simulink model "regcontrol_model_3ph"  (R2018b)
settings: Solver=VariableStepAuto  StartTime=0.0  StopTime=10.0  RelTol=1e-3
values from neighbouring files (symbols this model uses):
  BandWidth = Simulink.Parameter    [start.m]
  BaseVoltage = Simulink.Parameter    [start.m]
  CogenEnabled = false    [regcontrol_emulator.m]    (also in start.m = Simulink.Parameter)
  ElementTerminal = 0    [start.m]
  FPTphase = Simulink.Parameter(FPTphases.DEFAULT)    [regcontrol_emulator.m]    (also in start.m = 1)
  InCogenMode = false    [regcontrol_emulator.m]
  InReverseMode = false    [regcontrol_emulator.m]
  IsReversible = Simulink.Parameter    [start.m]
  LastHandle = RecentExecuted(1,NewCtrlQueueFields.Handle, end)    [LogEvent_1ph.m]    (also in LogEvent_1ph_old.m)
  LDC_Z = Simulink.Parameter    [start.m]
  MaxTap = 1.10    (= 1.1)    [Transformer.m]
  MinTap = 0.90    (= 0.9)    [Transformer.m]
  PTratio = Simulink.Parameter    [start.m]
  R = 0    [start.m]
  RevBand = Simulink.Parameter    [start.m]
  RevVreg = Simulink.Parameter    [start.m]
  TapLimitPerChange = Simulink.Parameter    [start.m]
  UsingRegulatedBus = Simulink.Parameter    [start.m]
  Vlimit = Simulink.Parameter    [start.m]
  Vreg = Simulink.Parameter    [start.m]
  X = 0    [start.m]
undefined symbols (not defined in the file or in its folder): Armed, ControlledTransformerConnection, ControlledTransformerCurrents, ControlledTransformerPowers, ControlledTransformerVoltages, CTRating, DeltaDirection, IsInverseTime, LastQueue, LookingForward, m, n, NumConductors, NumPhases, PresentTap, RevBackHandle, RevDelay, ReversePending, RevHandle, revLDC_Z, RevPowerThreshold, revR, revX, TapDelay, TapIncrement, TapWinding, TimeDelay, TimeInSec, VTerminal
(part 1 of 4)
settings Model: Creator=Michael Girbino  LastModifiedBy=Michael Girbino
settings DebuggingCC: LibraryContextMissingDiagnostic=none
settings SFSimCC: SimUseLocalCustomCode=off
settings RTWCC: RTWUseLocalCustomCode=off
settings CodeAppCC: StateflowObjectComments=on

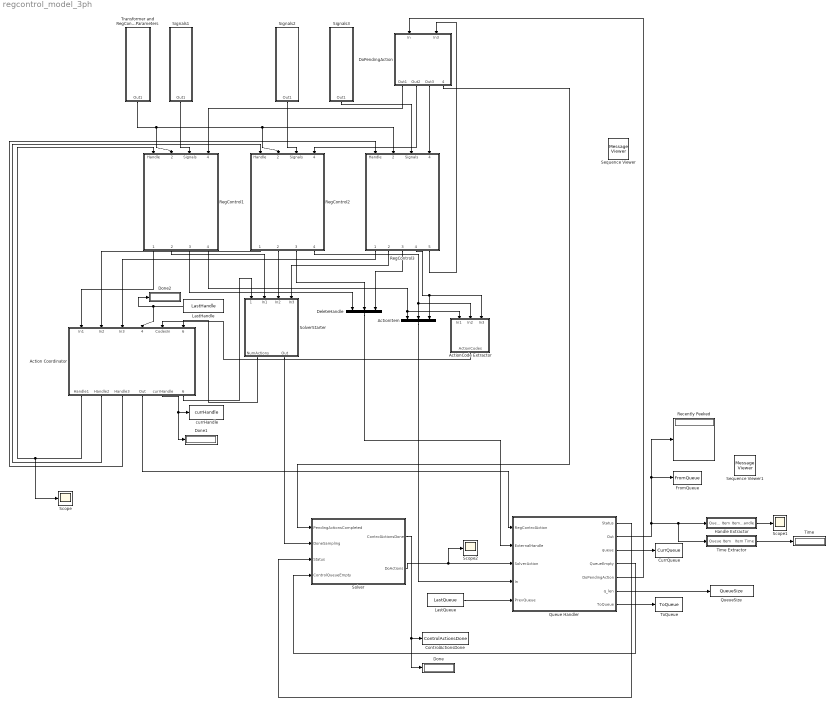
== system regcontrol_model_3ph ==
  Action Coordinator : Stateflow chart  TreatAsAtomicUnit=on
  "ActionCode Extractor " : Subsystem
  ActionItem : Concatenate  NumInputs=3  Mode=Multidimensional array  ConcatenateDimension=2
  ControlActionsDone : ToWorkspace  VariableName=ControlActionsDone  SaveFormat=Timeseries  SampleTime=-1
      settings: MaxDataPoints=1
  CurrQueue : ToWorkspace  VariableName=CurrQueue  SaveFormat=Structure With Time  SampleTime=1
  DeleteHandle : Mux  Inputs=3
  DoPendingAction : Stateflow chart  TreatAsAtomicUnit=on
  Done : Display
  Done1 : Display
  Done2 : Display
  FromQueue : ToWorkspace  VariableName=FromQueue  SaveFormat=Structure With Time  SampleTime=1
  Handle Extractor : Subsystem
  LastHandle : Constant  Value=LastHandle
  LastQueue : Constant  Value=LastQueue  VectorParams1D=off  OutDataTypeStr=double
  Queue Handler : Stateflow chart  TreatAsAtomicUnit=on
  QueueSize : ToWorkspace  VariableName=QueueSize  SaveFormat=Timeseries  SampleTime=-1
      settings: MaxDataPoints=1
  Recently Peeked : Display
  RegControl1 : Subsystem
  RegControl2 : Subsystem
  RegControl3 : Subsystem
  Scope : Scope
  Scope1 : Scope
  Scope2 : Scope
  Sequence Viewer : MessageViewer
  Sequence Viewer1 : MessageViewer
  Signals1 : Subsystem
  Signals2 : Subsystem
  Signals3 : Subsystem
  Solver : Stateflow chart  TreatAsAtomicUnit=on
  SolverStarter : Stateflow chart  TreatAsAtomicUnit=on
  Time : Display
  Time Extractor : Subsystem
  ToQueue : ToWorkspace  VariableName=ToQueue  SaveFormat=Structure With Time  SampleTime=-1
      settings: MaxDataPoints=1
  Transformer and RegControl Parameters : Subsystem
  currHandle : ToWorkspace  VariableName=currHandle  SaveFormat=Timeseries  SampleTime=-1
      settings: MaxDataPoints=1
  wires:
  Signals1/1(Out1) -> RegControl1/3(Signals)
  Transformer and RegControl Parameters/1(Out1) -> RegControl3/2(Equipment), RegControl2/2(Equipment), RegControl1/2(Equipment)
  DoPendingAction/1(Out1) -> RegControl1/4(DoPendingAction)
  DoPendingAction/2(Out2) -> RegControl2/4(DoPendingAction)
  DoPendingAction/3(Out3) -> RegControl3/4(DoPendingAction)
  RegControl1/1(DoActions) -> Action Coordinator/1(In1)
  RegControl2/1(DoActions) -> Action Coordinator/2(In2)
  RegControl3/1(DoActions) -> Action Coordinator/3(In3)
  RegControl1/2(DoneSampling) -> SolverStarter/2(In1)
  RegControl2/2(DoneSampling) -> SolverStarter/3(In2)
  RegControl3/2(DoneSampling) -> SolverStarter/4(In3)
  RegControl1/3(DeleteHandle) -> DeleteHandle/1
  RegControl2/3(DeleteHandle) -> DeleteHandle/2
  RegControl3/3(DeleteHandle) -> DeleteHandle/3
  RegControl2/4(ActionItem) -> "ActionCode Extractor "/2(In2), ActionItem/2
  RegControl3/4(ActionItem) -> "ActionCode Extractor "/3(In3), ActionItem/3
  DeleteHandle/1 -> Queue Handler/2(ExternalHandle)
  Queue Handler/6(q_len) -> QueueSize/1
  Solver/2(DoActions) -> Scope2/1, Queue Handler/3(SolverAction)
  Handle Extractor/1(Item Handle) -> Scope1/1
  Action Coordinator/4(Out) -> Queue Handler/1(RegControlAction)
  SolverStarter/2(Out) -> Solver/2(DoneSampling)
  Queue Handler/2(Out) -> Time Extractor/1(Queue Item), Handle Extractor/1(Queue Item), FromQueue/1, Recently Peeked/1
  Queue Handler/5(DoPendingAction) -> DoPendingAction/1(In)
  Queue Handler/4(QueueEmpty) -> Solver/4(ControlQueueEmpty)
  Time Extractor/1(Item Time) -> Time/1
  Queue Handler/3(queue) -> CurrQueue/1
  LastQueue/1 -> Queue Handler/5(PrevQueue)
  Solver/1(ControlActionsDone) -> Done/1, ControlActionsDone/1
  ActionItem/1 -> Queue Handler/4(In)
  Queue Handler/1(Status) -> Solver/3(Status)
  Signals2/1(Out1) -> RegControl2/3(Signals)
  Signals3/1(Out1) -> RegControl3/3(Signals)
  Action Coordinator/5(currHandle) -> Done1/1, currHandle/1
  LastHandle/1 -> Done2/1, Action Coordinator/4(LastHandle)
  Action Coordinator/1(Handle1) -> Scope/1, RegControl1/1(Handle)
  Action Coordinator/2(Handle2) -> RegControl2/1(Handle)
  Action Coordinator/3(Handle3) -> RegControl3/1(Handle)
  Queue Handler/7(ToQueue) -> ToQueue/1
  "ActionCode Extractor "/1(ActionCodes) -> Action Coordinator/5(CodesIn)
  RegControl1/4(ActionItem) -> "ActionCode Extractor "/1(In1), ActionItem/1
  Action Coordinator/6(ActionsDone) -> SolverStarter/1(ActionsDone)
  SolverStarter/1(NumActions) -> Action Coordinator/6(NumActions)
  DoPendingAction/4(PendingActionsCompleted) -> Solver/1(PendingActionsCompleted)
  RegControl3/5(PendingActionCompleted) -> DoPendingAction/2(In3)

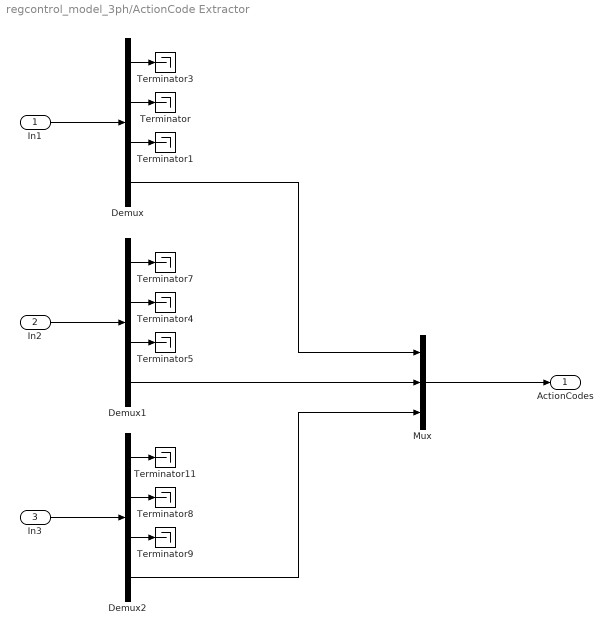
== system regcontrol_model_3ph/ActionCode Extractor  ==
  In1 : Inport
  In2 : Inport  Port=2
  In3 : Inport  Port=3
  Demux : Demux
  Demux1 : Demux
  Demux2 : Demux
  Mux : Mux  Inputs=3
  Terminator{,1,3..5,7..9,11} (9 alike) : Terminator
  ActionCodes : Outport
  wires:
  In1/1 -> Demux/1
  Demux/3 -> Terminator1/1
  Demux/4 -> Mux/1
  Demux/1 -> Terminator3/1
  Demux/2 -> Terminator/1
  Demux1/2 -> Terminator4/1
  Demux1/1 -> Terminator7/1
  Demux1/4 -> Mux/2
  Demux1/3 -> Terminator5/1
  In2/1 -> Demux1/1
  In3/1 -> Demux2/1
  Demux2/3 -> Terminator9/1
  Demux2/4 -> Mux/3
  Demux2/1 -> Terminator11/1
  Demux2/2 -> Terminator8/1
  Mux/1 -> ActionCodes/1

== system regcontrol_model_3ph/Handle Extractor ==
  Queue Item : Inport
  Demux : Demux  Outputs=6
  Terminator{,1..4} (5 alike) : Terminator
  Item Handle : Outport
  wires:
  Queue Item/1 -> Demux/1
  Demux/4 -> Terminator2/1
  Demux/3 -> Terminator1/1
  Demux/5 -> Terminator3/1
  Demux/1 -> Item Handle/1
  Demux/2 -> Terminator/1
  Demux/6 -> Terminator4/1

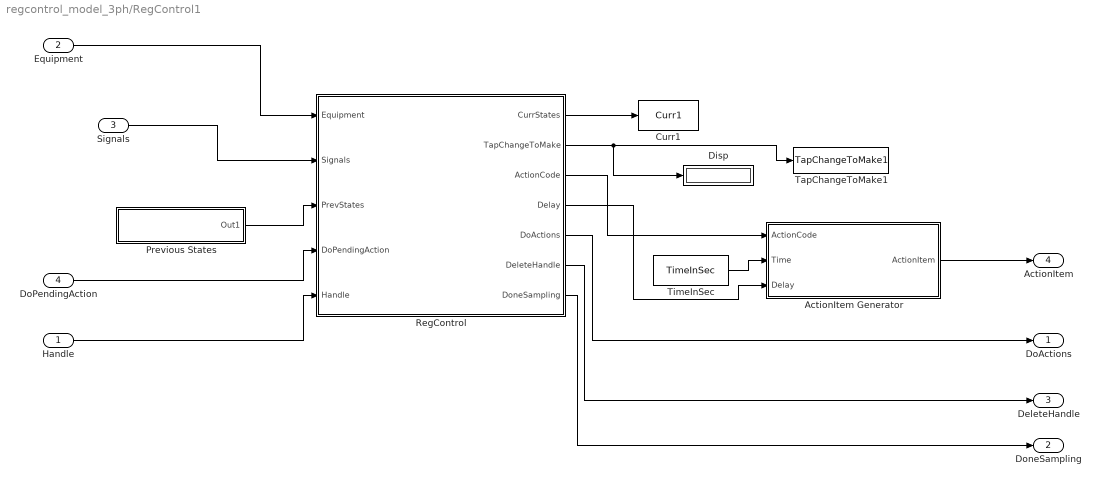
== system regcontrol_model_3ph/RegControl1 ==
  Handle : Inport
  Equipment : Inport  Port=2
  Signals : Inport  Port=3
  DoPendingAction : Inport  Port=4
  ActionItem Generator : Subsystem
  Curr1 : ToWorkspace  VariableName=Curr1  SaveFormat=Timeseries  SampleTime=-1
      settings: MaxDataPoints=1
  Disp : Display
  Previous States : Subsystem
  RegControl : Stateflow chart  TreatAsAtomicUnit=on
  TapChangeToMake1 : ToWorkspace  VariableName=TapChangeToMake1  SaveFormat=Timeseries  SampleTime=-1
      settings: MaxDataPoints=1
  TimeInSec : Constant  Value=TimeInSec  OutDataTypeStr=double
  DoActions : Outport
  DoneSampling : Outport  Port=2
  DeleteHandle : Outport  Port=3
  ActionItem : Outport  Port=4
  wires:
  RegControl/5(DoActions) -> DoActions/1
  RegControl/2(TapChangeToMake) -> Disp/1, TapChangeToMake1/1
  RegControl/4(Delay) -> ActionItem Generator/3(Delay)
  RegControl/3(ActionCode) -> ActionItem Generator/1(ActionCode)
  TimeInSec/1 -> ActionItem Generator/2(Time)
  ActionItem Generator/1(ActionItem) -> ActionItem/1
  RegControl/1(CurrStates) -> Curr1/1
  DoPendingAction/1 -> RegControl/4(DoPendingAction)
  Equipment/1 -> RegControl/1(Equipment)
  Signals/1 -> RegControl/2(Signals)
  RegControl/7(DoneSampling) -> DoneSampling/1
  Previous States/1(Out1) -> RegControl/3(PrevStates)
  RegControl/6(DeleteHandle) -> DeleteHandle/1
  Handle/1 -> RegControl/5(Handle)

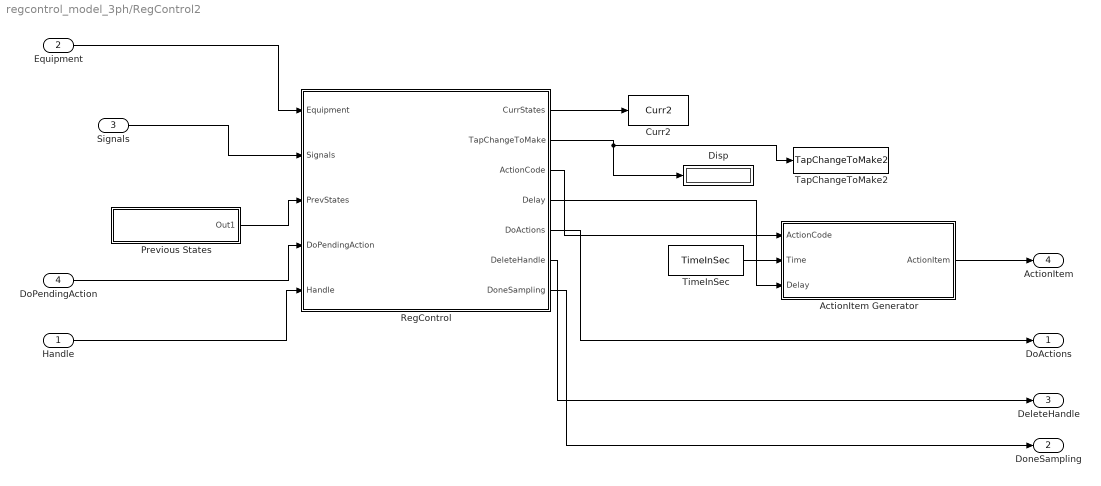
== system regcontrol_model_3ph/RegControl2 ==
  Handle : Inport
  Equipment : Inport  Port=2
  Signals : Inport  Port=3
  DoPendingAction : Inport  Port=4
  ActionItem Generator : Subsystem
  Curr2 : ToWorkspace  VariableName=Curr2  SaveFormat=Timeseries  SampleTime=-1
      settings: MaxDataPoints=1
  Disp : Display
  Previous States : Subsystem
  RegControl : Stateflow chart  TreatAsAtomicUnit=on
  TapChangeToMake2 : ToWorkspace  VariableName=TapChangeToMake2  SaveFormat=Timeseries  SampleTime=-1
      settings: MaxDataPoints=1
  TimeInSec : Constant  Value=TimeInSec  OutDataTypeStr=double
  DoActions : Outport
  DoneSampling : Outport  Port=2
  DeleteHandle : Outport  Port=3
  ActionItem : Outport  Port=4
  wires:
  RegControl/6(DeleteHandle) -> DeleteHandle/1
  Previous States/1(Out1) -> RegControl/3(PrevStates)
  RegControl/7(DoneSampling) -> DoneSampling/1
  Signals/1 -> RegControl/2(Signals)
  Equipment/1 -> RegControl/1(Equipment)
  DoPendingAction/1 -> RegControl/4(DoPendingAction)
  RegControl/1(CurrStates) -> Curr2/1
  ActionItem Generator/1(ActionItem) -> ActionItem/1
  TimeInSec/1 -> ActionItem Generator/2(Time)
  RegControl/3(ActionCode) -> ActionItem Generator/1(ActionCode)
  RegControl/4(Delay) -> ActionItem Generator/3(Delay)
  RegControl/2(TapChangeToMake) -> TapChangeToMake2/1, Disp/1
  RegControl/5(DoActions) -> DoActions/1
  Handle/1 -> RegControl/5(Handle)

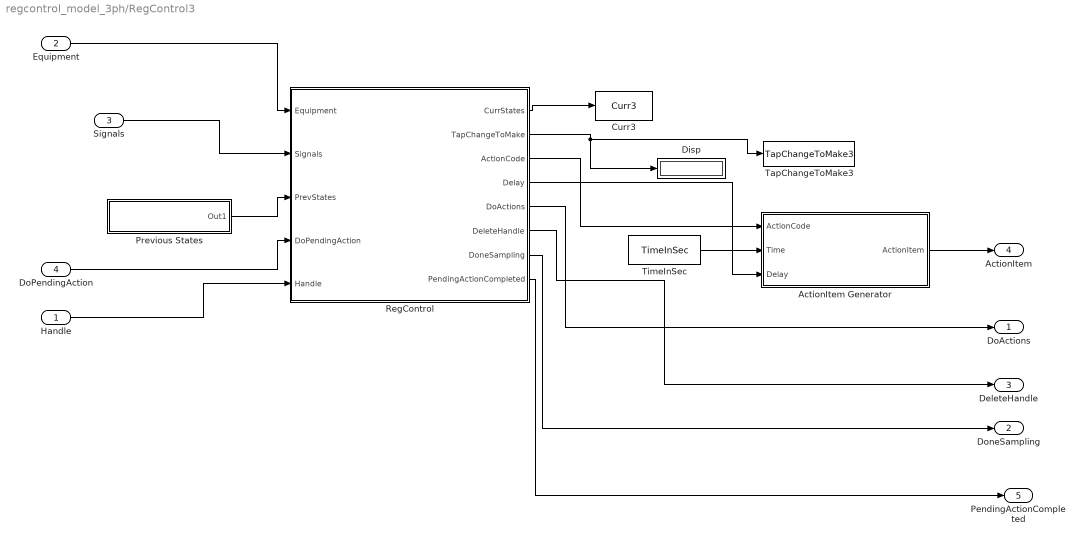
== system regcontrol_model_3ph/RegControl3 ==
  Handle : Inport
  Equipment : Inport  Port=2
  Signals : Inport  Port=3
  DoPendingAction : Inport  Port=4
  ActionItem Generator : Subsystem
  Curr3 : ToWorkspace  VariableName=Curr3  SaveFormat=Timeseries  SampleTime=-1
      settings: MaxDataPoints=1
  Disp : Display
  Previous States : Subsystem
  RegControl : Stateflow chart  TreatAsAtomicUnit=on
  TapChangeToMake3 : ToWorkspace  VariableName=TapChangeToMake3  SaveFormat=Timeseries  SampleTime=-1
      settings: MaxDataPoints=1
  TimeInSec : Constant  Value=TimeInSec  OutDataTypeStr=double
  DoActions : Outport
  DoneSampling : Outport  Port=2
  DeleteHandle : Outport  Port=3
  ActionItem : Outport  Port=4
  PendingActionCompleted : Outport  Port=5
  wires:
  RegControl/5(DoActions) -> DoActions/1
  RegControl/2(TapChangeToMake) -> Disp/1, TapChangeToMake3/1
  RegControl/4(Delay) -> ActionItem Generator/3(Delay)
  RegControl/3(ActionCode) -> ActionItem Generator/1(ActionCode)
  TimeInSec/1 -> ActionItem Generator/2(Time)
  ActionItem Generator/1(ActionItem) -> ActionItem/1
  RegControl/1(CurrStates) -> Curr3/1
  DoPendingAction/1 -> RegControl/4(DoPendingAction)
  Equipment/1 -> RegControl/1(Equipment)
  Signals/1 -> RegControl/2(Signals)
  RegControl/7(DoneSampling) -> DoneSampling/1
  Previous States/1(Out1) -> RegControl/3(PrevStates)
  RegControl/6(DeleteHandle) -> DeleteHandle/1
  Handle/1 -> RegControl/5(Handle)
  RegControl/8(PendingActionCompleted) -> PendingActionCompleted/1

== system regcontrol_model_3ph/Signals1 ==
  Bus Creator1 : BusCreator  Inputs=4  OutDataTypeStr=Bus: SignalBus
      settings: InheritFromInputs=off
  ControlledTransformerCurrents : Constant  Value=ControlledTransformerCurrents(:,1)
  ControlledTransformerPowers : Constant  Value=ControlledTransformerPowers(:,1)
  ControlledTransformerVoltages : Constant  Value=ControlledTransformerVoltages(:,1)
  VTerminal : Constant  Value=VTerminal(:,1)
  Out1 : Outport
  wires:
  Bus Creator1/1 -> Out1/1
  ControlledTransformerPowers/1 -> Bus Creator1/3
  ControlledTransformerVoltages/1 -> Bus Creator1/1
  ControlledTransformerCurrents/1 -> Bus Creator1/2
  VTerminal/1 -> Bus Creator1/4

== system regcontrol_model_3ph/Signals2 ==
  Bus Creator1 : BusCreator  Inputs=4  OutDataTypeStr=Bus: SignalBus
      settings: InheritFromInputs=off
  ControlledTransformerCurrents : Constant  Value=ControlledTransformerCurrents(:,2)
  ControlledTransformerPowers : Constant  Value=ControlledTransformerPowers(:,2)
  ControlledTransformerVoltages : Constant  Value=ControlledTransformerVoltages(:,2)
  VTerminal : Constant  Value=VTerminal(:,2)
  Out1 : Outport
  wires:
  ControlledTransformerCurrents/1 -> Bus Creator1/2
  ControlledTransformerPowers/1 -> Bus Creator1/3
  VTerminal/1 -> Bus Creator1/4
  ControlledTransformerVoltages/1 -> Bus Creator1/1
  Bus Creator1/1 -> Out1/1

== system regcontrol_model_3ph/Signals3 ==
  Bus Creator1 : BusCreator  Inputs=4  OutDataTypeStr=Bus: SignalBus
      settings: InheritFromInputs=off
  ControlledTransformerCurrents : Constant  Value=ControlledTransformerCurrents(:,3)
  ControlledTransformerPowers : Constant  Value=ControlledTransformerPowers(:,3)
  ControlledTransformerVoltages : Constant  Value=ControlledTransformerVoltages(:,3)
  VTerminal : Constant  Value=VTerminal(:,3)
  Out1 : Outport
  wires:
  ControlledTransformerCurrents/1 -> Bus Creator1/2
  ControlledTransformerPowers/1 -> Bus Creator1/3
  VTerminal/1 -> Bus Creator1/4
  ControlledTransformerVoltages/1 -> Bus Creator1/1
  Bus Creator1/1 -> Out1/1

== system regcontrol_model_3ph/Time Extractor ==
  Queue Item : Inport
  Demux : Demux  Outputs=6
  Terminator{,1..4} (5 alike) : Terminator
  Item Time : Outport
  wires:
  Demux/5 -> Terminator3/1
  Demux/3 -> Terminator1/1
  Demux/4 -> Terminator2/1
  Demux/1 -> Terminator/1
  Demux/2 -> Item Time/1
  Queue Item/1 -> Demux/1
  Demux/6 -> Terminator4/1

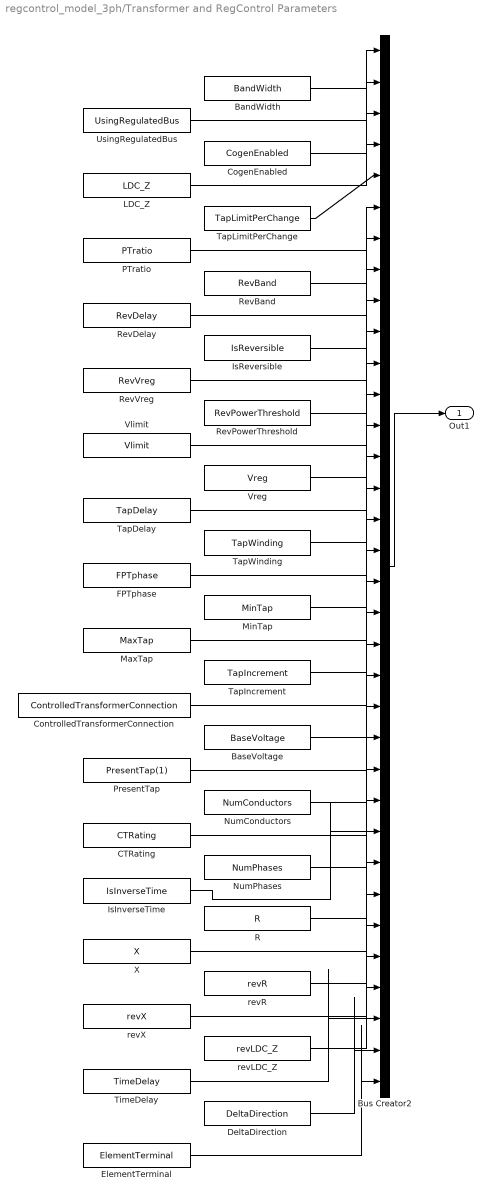
== system regcontrol_model_3ph/Transformer and RegControl Parameters ==
  BandWidth : Constant  Value=BandWidth
  BaseVoltage : Constant  Value=BaseVoltage
  Bus Creator2 : BusCreator  Inputs=34  OutDataTypeStr=Bus: EquipmentBus
      settings: InheritFromInputs=off
  CTRating : Constant  Value=CTRating
  CogenEnabled : Constant  Value=CogenEnabled
  ControlledTransformerConnection : Constant  Value=ControlledTransformerConnection
  DeltaDirection : Constant  Value=DeltaDirection
  ElementTerminal : Constant  Value=ElementTerminal
  FPTphase : Constant  Value=FPTphase
  IsInverseTime : Constant  Value=IsInverseTime
  IsReversible : Constant  Value=IsReversible
  LDC_Z : Constant  Value=LDC_Z
  MaxTap : Constant  Value=MaxTap
  MinTap : Constant  Value=MinTap
  NumConductors : Constant  Value=NumConductors
  NumPhases : Constant  Value=NumPhases
  PTratio : Constant  Value=PTratio
  PresentTap : Constant  Value=PresentTap(1)
  R : Constant  Value=R
  RevBand : Constant  Value=RevBand
  RevDelay : Constant  Value=RevDelay
  RevPowerThreshold : Constant  Value=RevPowerThreshold
  RevVreg : Constant  Value=RevVreg
  TapDelay : Constant  Value=TapDelay
  TapIncrement : Constant  Value=TapIncrement
  TapLimitPerChange : Constant  Value=TapLimitPerChange
  TapWinding : Constant  Value=TapWinding
  TimeDelay : Constant  Value=TimeDelay
  UsingRegulatedBus : Constant  Value=UsingRegulatedBus
  Vlimit : Constant  Value=Vlimit
  Vreg : Constant  Value=Vreg
  X : Constant  Value=X
  revLDC_Z : Constant  Value=revLDC_Z
  revR : Constant  Value=revR
  revX : Constant  Value=revX
  Out1 : Outport
  wires:
  UsingRegulatedBus/1 -> Bus Creator2/2
  BandWidth/1 -> Bus Creator2/1
  TapWinding/1 -> Bus Creator2/15
  TapDelay/1 -> Bus Creator2/14
  Vreg/1 -> Bus Creator2/13
  Vlimit/1 -> Bus Creator2/12
  RevPowerThreshold/1 -> Bus Creator2/11
  RevVreg/1 -> Bus Creator2/10
  IsReversible/1 -> Bus Creator2/9
  RevDelay/1 -> Bus Creator2/8
  RevBand/1 -> Bus Creator2/7
  PTratio/1 -> Bus Creator2/6
  TapLimitPerChange/1 -> Bus Creator2/5
  LDC_Z/1 -> Bus Creator2/4
  CogenEnabled/1 -> Bus Creator2/3
  Bus Creator2/1 -> Out1/1
  FPTphase/1 -> Bus Creator2/16
  MinTap/1 -> Bus Creator2/17
  MaxTap/1 -> Bus Creator2/18
  TapIncrement/1 -> Bus Creator2/19
  ControlledTransformerConnection/1 -> Bus Creator2/20
  BaseVoltage/1 -> Bus Creator2/21
  PresentTap/1 -> Bus Creator2/22
  NumConductors/1 -> Bus Creator2/23
  CTRating/1 -> Bus Creator2/24
  NumPhases/1 -> Bus Creator2/25
  revLDC_Z/1 -> Bus Creator2/31
  revX/1 -> Bus Creator2/30
  revR/1 -> Bus Creator2/29
  X/1 -> Bus Creator2/28
  R/1 -> Bus Creator2/27
  IsInverseTime/1 -> Bus Creator2/26
  TimeDelay/1 -> Bus Creator2/32
  DeltaDirection/1 -> Bus Creator2/33
  ElementTerminal/1 -> Bus Creator2/34

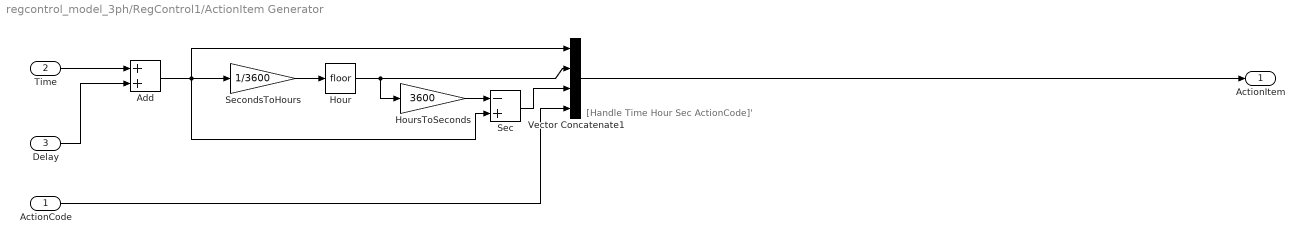
== system regcontrol_model_3ph/RegControl1/ActionItem Generator ==
  note: [Handle Time Hour Sec ActionCode]'
  ActionCode : Inport
  Time : Inport  Port=2
  Delay : Inport  Port=3
  Add : Sum
  Hour : Rounding
  HoursToSeconds : Gain  Gain=3600
  Sec : Sum  Inputs=-+
  SecondsToHours : Gain  Gain=1/3600
  Vector Concatenate1 : Concatenate  NumInputs=4
  ActionItem : Outport
  wires:
  Time/1 -> Add/1
  Hour/1 -> Vector Concatenate1/2, HoursToSeconds/1
  SecondsToHours/1 -> Hour/1
  Vector Concatenate1/1 -> ActionItem/1
  HoursToSeconds/1 -> Sec/1
  Sec/1 -> Vector Concatenate1/3
  ActionCode/1 -> Vector Concatenate1/4
  Delay/1 -> Add/2
  Add/1 -> Vector Concatenate1/1, Sec/2, SecondsToHours/1

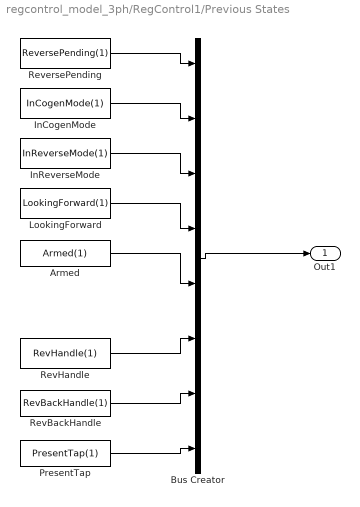
== system regcontrol_model_3ph/RegControl1/Previous States ==
  Armed : Constant  Value=Armed(1)
  Bus Creator : BusCreator  Inputs=8  OutDataTypeStr=Bus: StatesBus
      settings: InheritFromInputs=off
  InCogenMode : Constant  Value=InCogenMode(1)
  InReverseMode : Constant  Value=InReverseMode(1)
  LookingForward : Constant  Value=LookingForward(1)
  PresentTap : Constant  Value=PresentTap(1)
  RevBackHandle : Constant  Value=RevBackHandle(1)
  RevHandle : Constant  Value=RevHandle(1)
  ReversePending : Constant  Value=ReversePending(1)
  Out1 : Outport
  wires:
  Bus Creator/1 -> Out1/1
  ReversePending/1 -> Bus Creator/1
  InCogenMode/1 -> Bus Creator/2
  InReverseMode/1 -> Bus Creator/3
  LookingForward/1 -> Bus Creator/4
  Armed/1 -> Bus Creator/5
  RevHandle/1 -> Bus Creator/6
  RevBackHandle/1 -> Bus Creator/7
  PresentTap/1 -> Bus Creator/8

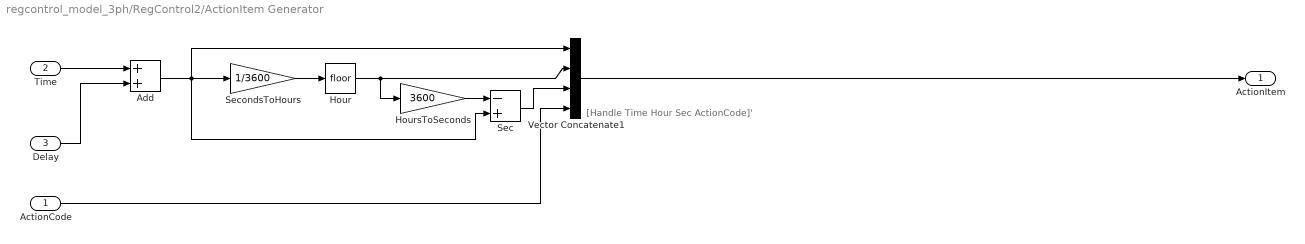
== system regcontrol_model_3ph/RegControl2/ActionItem Generator ==
  note: [Handle Time Hour Sec ActionCode]'
  ActionCode : Inport
  Time : Inport  Port=2
  Delay : Inport  Port=3
  Add : Sum
  Hour : Rounding
  HoursToSeconds : Gain  Gain=3600
  Sec : Sum  Inputs=-+
  SecondsToHours : Gain  Gain=1/3600
  Vector Concatenate1 : Concatenate  NumInputs=4
  ActionItem : Outport
  wires:
  Delay/1 -> Add/2
  Add/1 -> Vector Concatenate1/1, Sec/2, SecondsToHours/1
  HoursToSeconds/1 -> Sec/1
  SecondsToHours/1 -> Hour/1
  Hour/1 -> Vector Concatenate1/2, HoursToSeconds/1
  Vector Concatenate1/1 -> ActionItem/1
  Sec/1 -> Vector Concatenate1/3
  Time/1 -> Add/1
  ActionCode/1 -> Vector Concatenate1/4

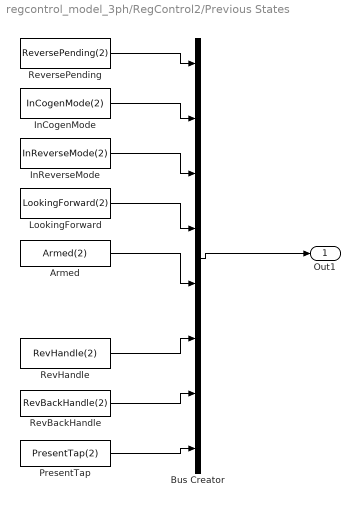
== system regcontrol_model_3ph/RegControl2/Previous States ==
  Armed : Constant  Value=Armed(2)
  Bus Creator : BusCreator  Inputs=8  OutDataTypeStr=Bus: StatesBus
      settings: InheritFromInputs=off
  InCogenMode : Constant  Value=InCogenMode(2)
  InReverseMode : Constant  Value=InReverseMode(2)
  LookingForward : Constant  Value=LookingForward(2)
  PresentTap : Constant  Value=PresentTap(2)
  RevBackHandle : Constant  Value=RevBackHandle(2)
  RevHandle : Constant  Value=RevHandle(2)
  ReversePending : Constant  Value=ReversePending(2)
  Out1 : Outport
  wires:
  Bus Creator/1 -> Out1/1
  RevHandle/1 -> Bus Creator/6
  RevBackHandle/1 -> Bus Creator/7
  InReverseMode/1 -> Bus Creator/3
  Armed/1 -> Bus Creator/5
  InCogenMode/1 -> Bus Creator/2
  ReversePending/1 -> Bus Creator/1
  PresentTap/1 -> Bus Creator/8
  LookingForward/1 -> Bus Creator/4

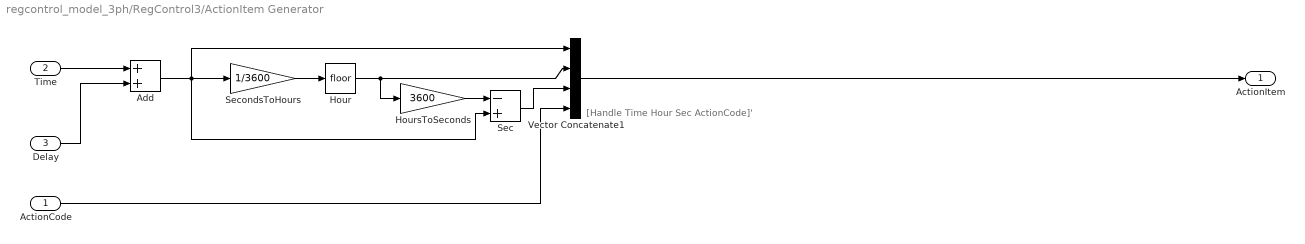
== system regcontrol_model_3ph/RegControl3/ActionItem Generator ==
  note: [Handle Time Hour Sec ActionCode]'
  ActionCode : Inport
  Time : Inport  Port=2
  Delay : Inport  Port=3
  Add : Sum
  Hour : Rounding
  HoursToSeconds : Gain  Gain=3600
  Sec : Sum  Inputs=-+
  SecondsToHours : Gain  Gain=1/3600
  Vector Concatenate1 : Concatenate  NumInputs=4
  ActionItem : Outport
  wires:
  Delay/1 -> Add/2
  Add/1 -> Vector Concatenate1/1, Sec/2, SecondsToHours/1
  HoursToSeconds/1 -> Sec/1
  SecondsToHours/1 -> Hour/1
  Hour/1 -> Vector Concatenate1/2, HoursToSeconds/1
  Vector Concatenate1/1 -> ActionItem/1
  Sec/1 -> Vector Concatenate1/3
  Time/1 -> Add/1
  ActionCode/1 -> Vector Concatenate1/4

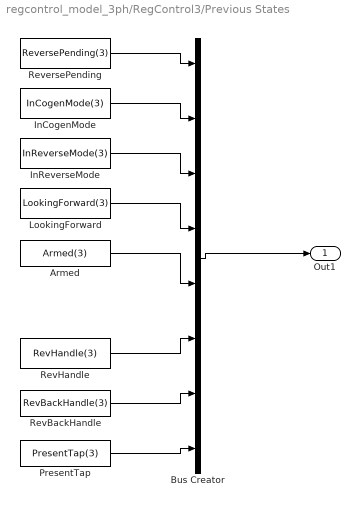
== system regcontrol_model_3ph/RegControl3/Previous States ==
  Armed : Constant  Value=Armed(3)
  Bus Creator : BusCreator  Inputs=8  OutDataTypeStr=Bus: StatesBus
      settings: InheritFromInputs=off
  InCogenMode : Constant  Value=InCogenMode(3)
  InReverseMode : Constant  Value=InReverseMode(3)
  LookingForward : Constant  Value=LookingForward(3)
  PresentTap : Constant  Value=PresentTap(3)
  RevBackHandle : Constant  Value=RevBackHandle(3)
  RevHandle : Constant  Value=RevHandle(3)
  ReversePending : Constant  Value=ReversePending(3)
  Out1 : Outport
  wires:
  Bus Creator/1 -> Out1/1
  RevHandle/1 -> Bus Creator/6
  RevBackHandle/1 -> Bus Creator/7
  InReverseMode/1 -> Bus Creator/3
  Armed/1 -> Bus Creator/5
  InCogenMode/1 -> Bus Creator/2
  ReversePending/1 -> Bus Creator/1
  PresentTap/1 -> Bus Creator/8
  LookingForward/1 -> Bus Creator/4

== stateflow chart regcontrol_model_3ph/RegControl2/RegControl ==
  settings: enableNonTerminalStates=1
  state Sampling [parallel]
    settings: executionOrder=1
    state DetermineReversePendingLookingForward
      state CorrectFalseReversePending
        en:
        if FwdPower < (-1*RevPowerThreshold)
        ReversePending = true;
        Push(ActionCodes.ACTION_REVERSE, ...
        RevDelay);
        % set flag requesting an update to RevHandle:
        UpdateRevHandle = true;
        end
      state CorrectTrueReversePending
        en:
        if FwdPower >= (-1*RevPowerThreshold)
        DeleteHandle = RevHandle;
        ReversePending = false;
        DoActions.data = QueueActions.DELETE;
        DoneSampling.data = uint8(DoneMsg.QUEUE_ACTION);
        send(DoActions);
        RevHandle = 0;
        end
      state Finished
        en: GET_VOLTAGE = true;
      (default) -> (junction 599) : {FwdPower = ...
          | -1*real( sum( ControlledTransformerPower((TerminalOffset+1):...
          | (TerminalOffset+NumConductors)) ) );}
          | % Should we reverse?
      (junction 599) -> Sampling.DetermineReversePendingLookingForward.CorrectFalseReversePending [order 1] : [~ReversePending]
      (junction 599) -> (junction 646) [order 2]
      Sampling.DetermineReversePendingLookingForward.CorrectFalseReversePending -> (junction 646)
      (junction 646) -> (junction 594)
      (junction 594) -> Sampling.DetermineReversePendingLookingForward.CorrectTrueReversePending [order 1] : [ReversePending]
      (junction 594) -> (junction 654) [order 2]
      Sampling.DetermineReversePendingLookingForward.CorrectTrueReversePending -> (junction 654)
      (junction 654) -> Sampling.DetermineReversePendingLookingForward.Finished
    state DetermineReversePendingLookingReverseOrCogen
      state CorrectFalseReversePending
        en:
        if FwdPower > RevPowerThreshold
        ReversePending = true;
        % push Reverse Back action to switch back:
        Push(ActionCodes.ACTION_REVERSE, ...
        RevDelay);
        % set flag requesting updated RevBackHandle:
        UpdateRevBackHandle = true;
        end
      state CorrectTrueReversePending
        en:
        if FwdPower <= RevPowerThreshold
        DeleteHandle = RevBackHandle;
        ReversePending = false;
        % delete Reverse Back action:
        DoActions.data = QueueActions.DELETE;
        DoneSampling.data = uint8(DoneMsg.QUEUE_ACTION);
        send(DoActions);
        RevBackHandle = 0;
        end
      state Finished
        en: REV_NEUTRAL = true;
      (default) -> (junction 620) : {FwdPower = ...
          | -1*real( sum( ControlledTransformerPower((TerminalOffset+1):...
          | (TerminalOffset+NumConductors)) ) );}
          | % If reversed, check if power is back in forward direction
      (junction 620) -> Sampling.DetermineReversePendingLookingReverseOrCogen.CorrectFalseReversePending [order 1] : [~ReversePending]
      (junction 620) -> (junction 621) [order 2]
      Sampling.DetermineReversePendingLookingReverseOrCogen.CorrectFalseReversePending -> (junction 621)
      (junction 621) -> (junction 624)
      (junction 624) -> Sampling.DetermineReversePendingLookingReverseOrCogen.CorrectTrueReversePending [order 1] : [ReversePending]
      (junction 624) -> (junction 650) [order 2]
      Sampling.DetermineReversePendingLookingReverseOrCogen.CorrectTrueReversePending -> (junction 650)
      (junction 650) -> Sampling.DetermineReversePendingLookingReverseOrCogen.Finished
    state ReverseNeutralCase
      state Finished
        en:
        GET_VOLTAGE = true;
      state ReverseNeutralTapChange
        en:
        PendingTapChange = ...
        round( (1.0 - double(TapWinding)) / TapIncrement ) * TapIncrement;
        if PendingTapChange ~= 0.0 && ~Armed
        Push(ActionCodes.ACTION_TAPCHANGE, TapDelay);
        Armed = true;
        end
      state Exiting
        en: EXIT = true;
      (default) -> (junction 592)
      (junction 592) -> (junction 637) [order 1] : % tap change not specified as needed:
          | [~Armed]
      (junction 592) -> Sampling.ReverseNeutralCase.Finished [order 2]
      (junction 637) -> (junction 614) : {PendingTapChange = 0.0;}
      (junction 614) -> (junction 638) [order 1] : [abs(PresentTap - 1.0) < EPSILON]
      (junction 614) -> Exiting [order 2]
      (junction 638) -> ReverseNeutralTapChange
      ReverseNeutralTapChange -> (junction 649)
      (junction 649) -> Exiting
    state GetVoltage
      en:
      if UsingRegulatedBus
      GetRegulatedBusVoltage; % stores voltages in VBuffer
      else
      VBuffer = ControlledTransformerWindingVoltages((TerminalOffset+1):(TerminalOffset+NumPhases));
      end
      Vcontrol = GetControlVoltage; % operates on VBuffer
    state DetermineVlocalbus
      state Finished
        en: GET_VOLTAGEWLDC = true;
      (default) -> (junction 689)
      (junction 689) -> (junction 691) [order 1] : % Voltage limit for bus connected to regulated winding; default = 0.0 (inactive)
          | [VlimitActive]
      (junction 689) -> Sampling.DetermineVlocalbus.Finished [order 2] : {Vlocalbus = 0.0;}
      (junction 691) -> (junction 683)
      (junction 683) -> (junction 692) [order 1] : % when controlled transformer is different from LDC PTransformer
          | [UsingRegulatedBus]
      (junction 683) -> (junction 696) [order 2] : % controlled transformer is
          | % the LDC PTransformer
          | {Vlocalbus = abs(Vcontrol);}
      (junction 692) -> (junction 714) : {%ControlledTransformer.GetWindingVoltages(ElementTerminal, VBuffer);
          | Vlocalbus = abs( VBuffer(1) / PTRatio );}
      (junction 714) -> (junction 696)
      (junction 696) -> (junction 675)
      (junction 675) -> Sampling.DetermineVlocalbus.Finished
    state GetVoltageWithLDC
      state RX_LDCmode
        en:
        if InReverseMode || InCogenMode
        VLDC = complex(revR, revX) * ...
        complex( real(ILDC), imag(ILDC) );
        else
        VLDC = complex(R, X) * ...
        complex( real(ILDC), imag(ILDC) );
        end
        Vcontrol = Vcontrol + VLDC;
      state Z_LDCmode
        en:
        if InReverseMode || InCogenMode
        Vcontrol = abs(Vcontrol) - abs(ILDC) * revLDC_Z;
        else
        Vcontrol = abs(Vcontrol) - abs(ILDC) * LDC_Z;
        end
      state Finished
        en: GET_TEST_VALUES = true;
      (default) -> (junction 771) : {% Convert current to control current by CTRating:
          | ILDC = ControlledTransformerCurrents(TerminalOffset + ControlledPhase) / CTRating;}
      (junction 771) -> RX_LDCmode [order 1] : % Standard R, X LDC
          | [LDC_Z == 0.0]
      (junction 771) -> Z_LDCmode [order 2] : % Beckwith LDC_Z control mode
      RX_LDCmode -> (junction 872)
      Z_LDCmode -> Sampling.GetVoltageWithLDC.Finished
      (junction 872) -> Sampling.GetVoltageWithLDC.Finished
    state GetTestValues
      en:
      Vactual = abs(Vcontrol);
      if InReverseMode
      Vactual = Vactual / PresentTap;
      VregTest = RevVreg;
      BandTest = RevBandwidth;
      else
      VregTest = Vreg;
      BandTest = Bandwidth;
      end
    state DetermineTapChangeIsNeeded
      en:
      if abs(VregTest - Vactual) > BandTest/2.0
      TapChangeIsNeeded = true;
      else
      TapChangeIsNeeded = false;
      end
    state MakeTapChange
      state GetVboostFromVlimit
        en:
        if Vlocalbus > Vlimit
        Vboost = Vlimit - Vlocalbus;
        end
      state TapChangeUp
        en:
        if PresentTap < MaxTap
        Push(ActionCodes.ACTION_TAPCHANGE, ...
        ComputeTimeDelay(Vactual));
        Armed = true;
        end
      state TapChangeDown
        en:
        if PresentTap > MinTap
        Push(ActionCodes.ACTION_TAPCHANGE, ...
        ComputeTimeDelay(Vactual));
        Armed = true;
        end
      state Finished
        en: FINISHED = true;
      (default) -> (junction 720) : % compute tapchange:
          | {Vboost = VregTest - Vactual;}
      (junction 720) -> (junction 766) [order 1] : [VlimitActive]
      (junction 720) -> (junction 723) [order 2]
      (junction 766) -> GetVboostFromVlimit
      GetVboostFromVlimit -> (junction 724)
      (junction 724) -> (junction 723)
      (junction 723) -> (junction 728) : {% PU winding boost needed:
          | BoostNeeded = Vboost * PTRatio / BaseVoltage;
          | Increment = TapIncrement;
          | % quantize to an increment:
          | PendingTapChange = ...
          | round(BoostNeeded/Increment)*Increment;
          | }
      (junction 728) -> (junction 731) : % send initial tap change message to ControlQueue, add delay time to solution control queue:
      (junction 731) -> (junction 817) [order 1] : % only changes 1 tap at a time:
          | [PendingTapChange ~= 0.0 && ~Armed]
      (junction 731) -> Sampling.MakeTapChange.Finished [order 2]
      (junction 817) -> (junction 810) : % see of any tap change is possible in desired direction (not saturated):
      (junction 810) -> TapChangeUp [order 1] : % going up:
          | [PendingTapChange > 0.0]
      (junction 810) -> TapChangeDown [order 2]
      TapChangeUp -> (junction 819)
      TapChangeDown -> (junction 820)
      (junction 820) -> Sampling.MakeTapChange.Finished
      (junction 819) -> (junction 820)
    state Finished
      en:
      WriteStatesToOutput;
      send(DoneSampling);
    (default) -> (junction 822) : {AssignEquipmentToLocals;
        | AssignSignalsToLocals;
        | AssignStatesToLocals;}
    (junction 822) -> (junction 815) [order 1] : [TapLimitPerChange ~= 0]
    (junction 815) -> (junction 826)
    (junction 822) -> (junction 807) [order 2]
    (junction 826) -> (junction 823) [order 1] : [~UsingRegulatedBus]
    (junction 826) -> (junction 818) [order 2]
    (junction 823) -> (junction 787)
    (junction 787) -> (junction 832) [order 1] : [IsReversible || CogenEnabled]
    (junction 787) -> (junction 792) [order 2]
    (junction 832) -> (junction 828)
    (junction 828) -> DetermineReversePendingLookingForward [order 1] : [LookingForward && ~InCogenMode]
    (junction 828) -> DetermineReversePendingLookingReverseOrCogen [order 2]
    DetermineReversePendingLookingForward -> (junction 825) : [GET_VOLTAGE]
    DetermineReversePendingLookingReverseOrCogen -> (junction 844) : [REV_NEUTRAL]
    (junction 844) -> ReverseNeutralCase [order 1] : % mode for which tap change may be executed,
        | % but no reversal made:
        | [ReverseNeutral]
    (junction 844) -> (junction 806) [order 2]
    ReverseNeutralCase -> (junction 806) [order 2] : [GET_VOLTAGE]
    (junction 806) -> (junction 808)
    ReverseNeutralCase -> (junction 829) [order 1] : [EXIT]
    (junction 792) -> (junction 818)
    (junction 808) -> (junction 792)
    (junction 825) -> (junction 808)
    (junction 818) -> GetVoltage
    (junction 829) -> (junction 807)
    (junction 807) -> (junction 816)
    GetVoltage -> DetermineVlocalbus
    DetermineVlocalbus -> (junction 845) : [GET_VOLTAGEWLDC]
    (junction 845) -> GetVoltageWithLDC [order 1] : % line drop compensation, but not using regulated bus
        | [~UsingRegulatedBus && LDCActive]
    (junction 845) -> (junction 809) [order 2]
    GetVoltageWithLDC -> (junction 839) : [GET_TEST_VALUES]
    (junction 839) -> (junction 809)
    (junction 809) -> GetTestValues
    GetTestValues -> DetermineTapChangeIsNeeded
    DetermineTapChangeIsNeeded -> (junction 788)
    (junction 788) -> MakeTapChange [order 1] : [TapChangeIsNeeded]
    (junction 788) -> (junction 813) [order 2]
    MakeTapChange -> (junction 837) : [FINISHED]
    (junction 837) -> (junction 813)
    (junction 813) -> Sampling.Finished
    (junction 816) -> Sampling.Finished : {PendingTapChange = 0;}
  state Execution [parallel]
    settings: executionOrder=2
    state Asleep
    state ParseAction
      en: Code = DoPendingAction.data;
      discard(DoPendingAction);
      length(DoPendingAction);
    state MakingTapChange
      en:
      if PendingTapChange ~= 0
      TapChangeToMake = AtLeastOneTap(PendingTapChange);
      PendingTapChange = 0;
      Armed = false;
      end
    state Reversing
      state FlipCogen
        en:
        if InCogenMode
        InCogenMode = false;
        else
        InCogenMode = true;
        end
      state FlipReverse
        en:
        if InReverseMode
        InReverseMode = false;
        else
        InReverseMode = true;
        end
      state Finished
        en:
        ReversePending = false;
        EXIT_REVERSE = true;
      (default) -> (junction 229)
      (junction 229) -> (junction 230) [order 1] : [ReversePending]
      (junction 229) -> Execution.Reversing.Finished [order 2]
      (junction 230) -> (junction 242)
      (junction 242) -> (junction 238) [order 1] : [CogenEnabled]
      (junction 242) -> FlipReverse [order 2]
      (junction 238) -> FlipCogen : % Cogen mode takes precedence if present
      FlipReverse -> (junction 240)
      FlipCogen -> (junction 245)
      (junction 240) -> Execution.Reversing.Finished
      (junction 245) -> (junction 240)
    state Finished
      en: WriteStatesToOutput;
    (default) -> Execution.Asleep
    Execution.Asleep -> ParseAction : DoPendingAction
    ParseAction -> (junction 115)
    (junction 115) -> MakingTapChange [order 1] : [Code == ActionCodes.ACTION_TAPCHANGE]
    (junction 115) -> (junction 119) [order 2]
    MakingTapChange -> (junction 122)
    (junction 119) -> Reversing [order 1] : [Code == ActionCodes.ACTION_REVERSE]
    (junction 119) -> (junction 123) [order 2]
    Reversing -> (junction 122) : [EXIT_REVERSE]
    (junction 122) -> (junction 124)
    (junction 124) -> (junction 123)
    (junction 123) -> Execution.Finished
  state ChangeToMake = AtLeastOneTap(ProposedChange) [function]
    note: Called in STATIC mode
        | Changes 70% of the way but at least one tap, subject to maximum allowable tap change
    (default) -> (junction 283) : {NumTaps = floor(0.7 * abs(ProposedChange)/TapIncrement);}
    (junction 283) -> (junction 284) [order 1] : [NumTaps == 0]
    (junction 283) -> (junction 285) [order 2]
    (junction 284) -> (junction 286) : {NumTaps = 1.0;} % At least 1 tap
    (junction 286) -> (junction 285)
    (junction 285) -> (junction 293)
    (junction 293) -> (junction 290) [order 1] : [NumTaps > TapLimitPerChange]
    (junction 293) -> (junction 294) [order 2]
    (junction 290) -> (junction 295) : {NumTaps = double(TapLimitPerChange);} % Bound by maximum
    (junction 295) -> (junction 294)
    (junction 294) -> (junction 302) : {LastChange = NumTaps;}
    (junction 302) -> (junction 303) [order 1] : % Check sign on change:
        | [ProposedChange > 0]
    (junction 302) -> (junction 304) [order 2] : {ChangeToMake = ...
        | -1*double(NumTaps)*TapIncrement;
        | LastChange = -1*NumTaps;}
    (junction 303) -> (junction 305) : {ChangeToMake =...
        |  double(NumTaps)*TapIncrement;}
    (junction 305) -> (junction 304)
    (junction 304) -> (junction 306)
  state Result = GetControlVoltage [function]
    note: GetControlVoltage
        | Called when voltage is sampled from the same transformer whose taps are controlled.
        | Returns the voltage which will be used to decide tap changes. Also changes the ControlledPhase if it is different from FPTphase.
    note: FPTphase is max phase.
        |
        | VControl is taken from the phase with the greatest voltage.
        |
        | ControlledPhase becomes that phase.
    note: FPTphase is min phase.
        |
        | VControl is taken from the phase with the least voltage.
        |
        | ControlledPhase becomes that phase.
    (default) -> (junction 496)
    (junction 496) -> (junction 486) [order 1] : [FPTphase == uint8(FPTphases.MAXPHASE)]
        | % controlled phase is that with greatest |V|
    (junction 496) -> (junction 517) [order 2]
    (junction 486) -> (junction 523) : {ControlledPhase = 1;
        | % abs is equivalent to Cabs:
        | V = abs( VBuffer(ControlledPhase) );}
        | % Iteration through remaining phases:
    (junction 510) -> (junction 489) [order 1] : [ii <= NumPhases]
    (junction 489) -> (junction 485)
    (junction 523) -> (junction 510) : {ii = uint8(2);}
    (junction 485) -> (junction 515) [order 1] : [abs( VBuffer(ControlledPhase)) > V]
        | % if it's GREATER, make it the new V
    (junction 485) -> (junction 522) [order 2]
    (junction 515) -> (junction 516) : {V = abs( VBuffer(ii) );
        | ControlledPhase = ii;}
    (junction 487) -> (junction 510) : {ii = ii+1;}
    (junction 510) -> (junction 534) [order 2] : {Result = VBuffer(ControlledPhase) / PTRatio;
        | % Complex divided by real
        | }
    (junction 516) -> (junction 522)
    (junction 522) -> (junction 487)
    (junction 534) -> (junction 527)
    (junction 527) -> (junction 519)
    (junction 517) -> (junction 533) [order 1] : [FPTphase == uint8(FPTphases.MINPHASE)]
        | % controlled phase is that with least |V|
    (junction 533) -> (junction 535) : {ControlledPhase = 1;
        | % abs is equivalent to Cabs:
        | V = abs( VBuffer(ControlledPhase) );}
        | % Iteration through remaining phases:
    (junction 517) -> (junction 1027) [order 2] : % Default case: use specified phase,
        | % as long as it's feasible
    (junction 513) -> (junction 537) [order 1] : [ii <= NumPhases]
    (junction 537) -> (junction 488)
    (junction 535) -> (junction 513) : {ii = uint8(2);}
    (junction 1027) -> (junction 1028) [order 1] : [FPTphase > NumPhases]
    (junction 488) -> (junction 504) [order 1] : [abs( VBuffer(ControlledPhase)) < V]
        | % if it's LESS, make it the new V
    (junction 1027) -> (junction 1029) [order 2] : {FPTphase = max(FPTphase, 1);}
    (junction 1028) -> (junction 1030) : {FPTphase = 1;}
    (junction 488) -> (junction 514) [order 2]
    (junction 504) -> (junction 507) : {V = abs( VBuffer(ii) );
        | ControlledPhase = ii;}
    (junction 518) -> (junction 513) : {ii = ii+1;}
    (junction 513) -> (junction 536) [order 2] : {Result = VBuffer(ControlledPhase) / PTRatio;
        | % Complex divided by real
        | }
    (junction 507) -> (junction 514)
    (junction 514) -> (junction 518)
    (junction 1030) -> (junction 1029)
    (junction 1029) -> (junction 497) : {Result = VBuffer(FPTphase) / PTRatio;
        | ControlledPhase = FPTphase;}
    (junction 536) -> (junction 519)
    (junction 519) -> (junction 502)
    (junction 502) -> (junction 497)
    (junction 497) -> (junction 498)
  state Result = ComputeTimeDelay(Vavg) [function]
    (default) -> (junction 477)
    (junction 477) -> (junction 481) [order 1] : [IsInverseTime]
    (junction 477) -> (junction 482) [order 2] : % determines which regulator control will act first,
        | % default is 15s
        | {Result = TimeDelay;}
    (junction 481) -> (junction 483) : % TimeDelay is adjusted inversely proportional to
        | % the amount that voltage is outside the band,
        | % down to 10 percent of specified time delay
        | % (Further out of band = band - 1> less time delay)
        | {Result = TimeDelay / min(10.0, 2.0*abs(Vreg - Vavg)/Bandwidth);}
    (junction 483) -> (junction 482)
    (junction 482) -> (junction 474)
  state AssignEquipmentToLocals [function]
    (default) -> (junction 550) : {
        | BandWidth = Equipment.BandWidth;
        | UsingRegulatedBus = Equipment.UsingRegulatedBus;
        | CogenEnabled = Equipment.CogenEnabled;
        | LDC_Z = Equipment.LDC_Z;
        | TapLimitPerChange = Equipment.TapLimitPerChange;
        | PTRatio = Equipment.PTratio;
        | RevBand = Equipment.RevBand;
        | RevDelay = Equipment.RevDelay;
        | IsReversible = Equipment.IsReversible;
        | RevVreg = Equipment.RevVreg;
        | RevPowerThreshold = Equipment.RevPowerThreshold;
        | Vlimit = Equipment.Vlimit;
        | Vreg = Equipment.Vreg;
        | TapDelay = Equipment.TapDelay;
        | TapWinding = Equipment.TapWinding;
        | FPTphase = Equipment.FPTphase;
        |
        | MinTap = Equipment.MinTap;
        | MaxTap = Equipment.MaxTap;
        | TapIncrement = Equipment.TapIncrement;
        | ControlledTransformerConnection = Equipment.ControlledTransformerConnection;
        | BaseVoltage = Equipment.BaseVoltage;
        | NumConductors = Equipment.NumConductors;
        | NumPhases = Equipment.NumPhases;
        | CTRating = Equipment.CTRating;
        | IsInverseTime = Equipment.IsInverseTime;
        |
        | R = Equipment.R;
        | X = Equipment.X;
        | revR = Equipment.revR;
        | revX = Equipment.revX;
        | revLDC_Z = Equipment.revLDC_Z;
        | TimeDelay = Equipment.TimeDelay;
        |
        | % From Script:
        | TapWinding = Equipment.TapWinding;
        | TapIncrement = Equipment.TapIncrement;
        | TapDelay = Equipment.TapDelay;
        | CogenEnabled = Equipment.CogenEnabled;
        | % PresentTap = Equipment.PresentTap;
        | TapLimitPerChange = Equipment.TapLimitPerChange;
        | ElementTerminal = Equipment.ElementTerminal;
        | DeltaDirection = Equipment.DeltaDirection;
        | DoneSampling.data = uint8(DoneMsg.NO_ACTION);
        | }
    (junction 550) -> (junction 548) [order 1] : [R~=0 || X~=0 || LDC_Z ~=0]
    (junction 550) -> (junction 555) [order 2] : {LDCActive = false;}
    (junction 548) -> (junction 552) : {LDCActive = true;}
    (junction 552) -> (junction 555)
    (junction 555) -> (junction 547)
  state Push(CodeVal, DelayVal) [function]
    (default) -> (junction 1082) : {ActionCode = double(CodeVal);
        | Delay = DelayVal;
        | DoActions.data = QueueActions.PUSH;
        | DoneSampling.data = uint8(DoneMsg.QUEUE_ACTION);
        | send(DoActions);
        | }
  state UpdateStoredHandles [parallel]
    settings: executionOrder=3
    note: - Updates local copies of RevHandle and RevBackHAndle
        | - Only used when RegControl IsReversible
        | - Reversible implies that LDC has different parameters InReverseMode
    state Asleep
    state ReadHandle
      en: StoredHandle = Handle.data;
      discard(Handle);
    state Finished
      en: WriteStatesToOutput;
    (default) -> UpdateStoredHandles.Asleep
    UpdateStoredHandles.Asleep -> ReadHandle : Handle
    ReadHandle -> (junction 1103) [order 1] : [UpdateRevHandle == true]
    (junction 1103) -> (junction 1108) : {RevHandle = StoredHandle;
        | UpdateRevHandle = false;}
    ReadHandle -> (junction 1104) [order 2]
    (junction 1104) -> (junction 1105) [order 1] : [UpdateRevBackHandle == true]
    (junction 1104) -> UpdateStoredHandles.Finished [order 2]
    (junction 1105) -> (junction 1107) : {RevBackHandle = StoredHandle;
        | UpdateRevBackHandle = false;}
    (junction 1107) -> UpdateStoredHandles.Finished
    (junction 1108) -> (junction 1107)
  state AssignSignalsToLocals [function]
    (default) -> (junction 940) : {ControlledTransformerWindingVoltages = Signals.ControlledTransformerVoltages;
        | ControlledTransformerPower = Signals.ControlledTransformerPowers;
        | ControlledTransformerCurrents = Signals.ControlledTransformerCurrents;
        | VTerminal = Signals.VTerminal;
        |
        | TerminalOffset = NumConductors*(ElementTerminal - 1);
        | VBuffer = zeros(NumPhases, 1);}
  state AssignStatesToLocals [function]
    (default) -> (junction 943) : {ReversePending = PrevStates.ReversePending;
        | InCogenMode = PrevStates.InCogenMode;
        | InReverseMode = PrevStates.InReverseMode;
        | LookingForward = PrevStates.LookingForward;
        | Armed = PrevStates.Armed;
        | RevHandle = PrevStates.RevHandle;
        | RevBackHandle = PrevStates.RevBackHandle;
        | PresentTap = PrevStates.PresentTap;
        | }
  state GetRegulatedBusVoltage [function]
    (junction 989) -> (junction 998) [order 1] : [ii <= NumPhases]
    (default) -> (junction 989) : {ii = uint8(1);}
    (junction 998) -> (junction 1002)
    (junction 1002) -> (junction 991) [order 1] : [ControlledTransformerConnection == Connections.DELTA]
    (junction 1002) -> (junction 1015) [order 2]
    (junction 991) -> (junction 992) : {rotIdx = RotatePhases(ii, NumPhases, DeltaDirection);
        | VBuffer(ii) = VTerminal(TerminalOffset+ii) - ...
        | VTerminal(TerminalOffset+rotIdx);}
    (junction 1015) -> (junction 1007) [order 1] : [ControlledTransformerConnection == ...
        | Connections.WYE]
    (junction 1015) -> (junction 1017) [order 2]
    (junction 1007) -> (junction 990) : {VBuffer(ii) = VTerminal(TerminalOffset+ii);}
    (junction 997) -> (junction 989) : {ii = ii+1;}
    (junction 989) -> (junction 1005) [order 2]
    (junction 990) -> (junction 1017)
    (junction 992) -> (junction 990)
    (junction 1017) -> (junction 997)
  state WriteStatesToOutput [function]
    (default) -> (junction 947) : {CurrStates.ReversePending = ReversePending;
        | CurrStates.InCogenMode = InCogenMode;
        | CurrStates.InReverseMode = InReverseMode;
        | CurrStates.LookingForward = LookingForward;
        | CurrStates.Armed = Armed;
        | CurrStates.RevHandle = RevHandle;
        | CurrStates.RevBackHandle = RevBackHandle;
        | CurrStates.PresentTap = PresentTap;
        | }
  data: ProposedChange function_input; ChangeToMake function_output; NumTaps local double; Result function_output; Vavg function_input; Result function_output; CodeVal function_input; DelayVal function_input; idx function_input; newIdx function_output; NPhases function_input; DeltaDir function_input; CurrStates output Bus: StatesBus; Equipment input Bus: EquipmentBus; Signals input Bus: SignalBus; PrevStates input Bus: StatesBus; EXIT_REVERSE local boolean =false; InReverseMode local boolean =false; ReversePending local boolean =false; InCogenMode local boolean =false; DoPendingAction input double; TapWinding local uint8; TapIncrement local double; TapDelay local double; CogenEnabled local boolean =false; TapChangeToMake output double; PendingTapChange local double =double(0); TapLimitPerChange local uint8 =uint8(16); ActionCode output double; Delay output double =0; DoActions output Enum: QueueActions; DeleteHandle output uint8 size=[1] =uint8(0); DoneSampling output uint8 =uint8(0); Armed local boolean =false; PresentTap local double; Vactual local double =0; Vcontrol local double =complex(0); FPTphase local uint8 size=[1]; VBuffer local double size=[3 1]; NumPhases local uint8 size=[1]; ControlledPhase local uint8 size=[1] =uint8(1); PTRatio local double =60; IsInverseTime local boolean; TimeDelay local double; Vreg local double =120; Bandwidth local double =3; revR local double =0; RevVreg local double =120; revX local double =0; ControlledTransformerConnection local uint8 size=[1]; ControlledTransformerCurrents local double; ControlledTransformerPower local double; ControlledTransformerWindingVoltages local double size=[4 1]; CTRating local double; MaxTap local double; MinTap local double; Vlimit local double =0; RevDelay local double; revLDC_Z local double =0; RevPowerThreshold local double; RevBandwidth local double =3; ElementTerminal local uint8 size=[1] =uint8(1); LDCActive local boolean =false; VlimitActive local boolean =false; Increment local double =0; IsReversible local boolean =false; LookingForward local boolean =false; ReverseNeutral local boolean =false; NumConductors local uint8 size=[1]; BaseVoltage local double; UsingRegulatedBus local boolean =false; VLDC local double =complex(0); FINISHED local boolean =false; VregTest local double =0; BandTest local double =0; EXIT local boolean =false; ILDC local double =complex(0); Vboost local double =0; FwdPower local double =0; GET_TEST_VALUES local boolean =false; GET_VOLTAGE local boolean =false; GET_VOLTAGEWLDC local boolean =false; Vlocalbus local double =0; BoostNeeded local double =0; RevBackHandle local uint8 size=[1] =uint8(0); REV_NEUTRAL local boolean =false; TapChangeIsNeeded local boolean =false; LDC_Z local double =0; R local double =0; X local double =0; EPSILON local double =1.0e-12; RevHandle local uint8 size=[1] =uint8(0); LastChange local double; DeltaDirection local uint8; VTerminal local double size=[4 1]; TerminalOffset local uint8 =uint8(0); Code local double size=[1 1]; Handle input uint8; UpdateRevHandle local boolean =false; UpdateRevBackHandle local boolean =false; StoredHandle local uint8
  function newIdx = RotatePhases(idx, NPhases, DeltaDir):
    | function newIdx = RotatePhases(idx, NPhases, DeltaDir)
    |     dd = int8(1);
    |     
    |     switch(DeltaDir)
    |         case DeltaDirs.FORWARD
    |             dd = int8(1);
    |         case DeltaDirs.REVERSE
    |             dd = int8(-1);
    |     end
    | 
    |     newIdx = uint8( int8(idx) + dd );
    | 
    |     % make sure RotatedPhase is within limits:
    |     if NPhases > 2
    |         % Assumes 2 phase delta is open delta
    |         if newIdx > NPhases
    |             newIdx = uint8(1);
    |         elseif newIdx < 1
    |             newIdx = NPhases;
    |         end
    |     elseif newIdx < 1
    |         newIdx = uint8(3); % For 2-phase delta, next phase will be 3rd phase
    |     end
    | end
